simulink model "dyn_model"  (R2023b)
settings: Solver=VariableStepAuto  StartTime=0.0  StopTime=100.0  RelTol=1e-3
values from neighbouring files (symbols this model uses):
  A = double(A)    [dyn_model_mark.m]
  B = double(B)    [dyn_model_mark.m]
  C = [1 0 0 0 ... (first row only)    [dyn_model_mark.m]
  D = [0 ... (first row only)    [dyn_model_mark.m]
  g0 = 9.81    [dyn_model_mark.m]
  Ip = (mp*Lp^2)/12    (= 8.3205e-06)    [dyn_model_mark.m]
  Ir = (mr*(Lr/2)^2)/12    (= 1.42994791667e-05)    [dyn_model_mark.m]
  J = 4e-6    (= 4e-06)    [dyn_model_mark.m]
  k = 42e-3    (= 0.042)    [dyn_model_mark.m]
  La = 1.16e-3    (= 0.00116)    [dyn_model_mark.m]
  Lp = 0.129/2    (= 0.0645)    [dyn_model_mark.m]
  Lr = 0.085    [dyn_model_mark.m]
  mp = 0.024    [dyn_model_mark.m]
  mr = 0.095    [dyn_model_mark.m]
  param = [mr mp Lr Lp Ir Ip g0]'    [dyn_model_mark.m]
  Ra = 8.4    [dyn_model_mark.m]
undefined symbols (not defined in the file or in its folder): rot_pend
libraries: slpidlib x2, simulink_extras x2, simulink x2
settings Model: Creator=Mark  LastModifiedBy=Mark
settings OptimizationCC: BlockReduction=off  DefaultParameterBehavior=Inlined  BufferReuse=off

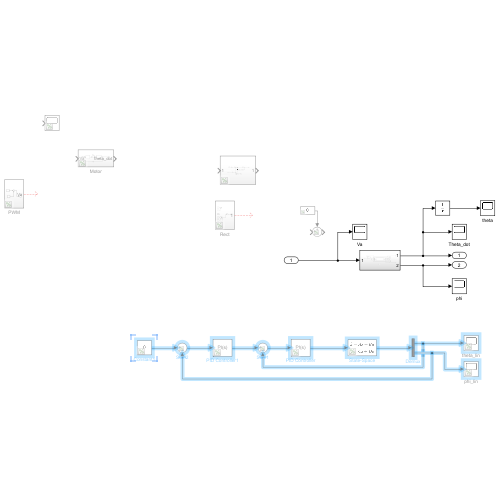
[thumbnail: Simulink's stored preview of the top-level diagram]
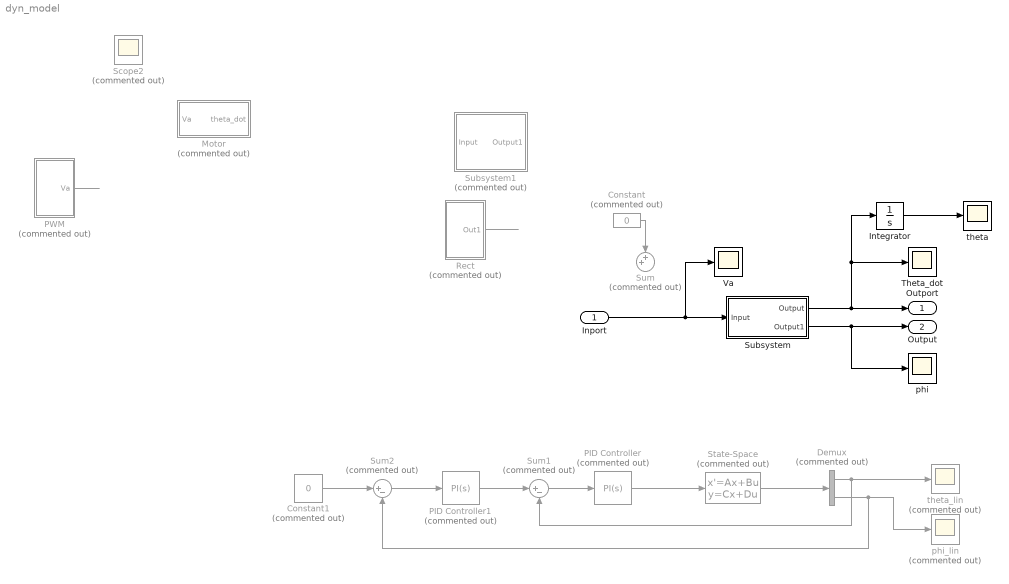
== system dyn_model ==
  Inport : Inport
  Constant : Constant  Commented=on  Value=0
  Constant1 : Constant  Commented=on  Value=0
  Demux : Demux  Commented=on  Outputs=2
  Integrator : Integrator
  Motor : Subsystem  Commented=on
  PID Controller : slpidlib/PID Controller  Commented=on  Controller=PI  Form=Parallel  TimeDomain=Continuous-time  UseExternalTs=off  SampleTime=-1  IntegratorMethod=Forward Euler  FilterMethod=Forward Euler  ControllerParametersSource=internal  P=1  I=1  UseKiTs=off  D=0  N=100  UseFilter=on  TunerSelectOption=Transfer Function Based (PID Tuner App)  InitialConditionSource=internal  InitialConditionForIntegrator=0  InitialConditionForFilter=0  DifferentiatorICPrevScaledInput=0  ExternalReset=none  TrackingMode=off  Kt=1  LimitOutput=off  SatLimitsSource=internal  UpperSaturationLimit=inf  LowerSaturationLimit=-inf  LinearizeAsGain=on  AntiWindupMode=none  Kb=1  LimitIntegrator=off  UpperIntegratorSaturationLimit=inf  LowerIntegratorSaturationLimit=-inf  POutMin=[]  POutMax=[]  IOutMin=[]  IOutMax=[]  DOutMin=[]  DOutMax=[]  NOutMin=[]  NOutMax=[]  SumOutMin=[]  SumOutMax=[]  SaturationOutMin=[]  SaturationOutMax=[]  PParamMin=[]  PParamMax=[]  IParamMin=[]  IParamMax=[]  DParamMin=[]  DParamMax=[]  NParamMin=[]  NParamMax=[]  KbParamMin=[]  KbParamMax=[]  KtParamMin=[]  KtParamMax=[]  KbOutMin=[]  KbOutMax=[]  KtOutMin=[]  KtOutMax=[]  IntegratorOutMin=[]  IntegratorOutMax=[]  FilterOutMin=[]  FilterOutMax=[]  SumI1OutMin=[]  SumI1OutMax=[]  SumI2OutMin=[]  SumI2OutMax=[]  SumI3OutMin=[]  SumI3OutMax=[]  SumI4OutMin=[]  SumI4OutMax=[]  SumDOutMin=[]  SumDOutMax=[]  DifferentiatorOutMin=[]  DifferentiatorOutMax=[]  FilterDiffOutCoefMin=[]  FilterDiffOutCoefMax=[]  ReciprocalOutMin=[]  ReciprocalOutMax=[]  SumDenOutMin=[]  SumDenOutMax=[]  SumNumOutMin=[]  SumNumOutMax=[]  DivideOutMin=[]  DivideOutMax=[]  UdiffTsProdOutMin=[]  UdiffTsProdOutMax=[]  NTsProdOutMin=[]  NTsProdOutMax=[]  UintegralTsProdOutMin=[]  UintegralTsProdOutMax=[]  UngainTsProdOutMin=[]  UngainTsProdOutMax=[]  ClampingZeroOutDataTypeStr=Inherit: Inherit via back propagation  ClampingZeroOutMin=[]  ClampingZeroOutMax=[]  FilterDenConstantOutDataTypeStr=Inherit: Inherit via back propagation  FilterDenConstantOutMin=[]  FilterDenConstantOutMax=[]  PCopyOutDataTypeStr=Inherit: Inherit via back propagation  PCopyOutMin=[]  PCopyOutMax=[]  NCopyOutDataTypeStr=Inherit: Inherit via back propagation  NCopyOutMin=[]  NCopyOutMax=[]  IntegratorContinuousStateAttributes=''  IntegratorStateMustResolveToSignalObject=off  IntegratorRTWStateStorageClass=Auto  FilterContinuousStateAttributes=''  FilterStateMustResolveToSignalObject=off  FilterRTWStateStorageClass=Auto  ParallelPVariant=InternalParameters  IdealPVariant=Disabled  IVariant=InternalParameters  DVariant=Disabled  IntegratorVariant=Continuous  SatVariant=Disabled  AWVariant=Passthrough  PCopyVariant=Disabled  TRVariant=Disabled  FdbkBlocksVariant=Forward  IdealPFdbkVariant=Disabled  SatFdbkVariant=Disabled  DerivativeFilterVariant=Disabled  NVariant=Disabled  NCopyVariant=Disabled_SignalSpec  FilterICVariant=Disabled  IntegratorICVariant=InternalICs  ExternalResetVariant=Disabled  TRSumVariant=Passthrough  SumFdbkVariant=Disabled  SumVariant=Sum_PI  TsampFilterVariant=InternalTs  TsampNgainVariant=Passthrough  TsampIntegralVariant=Disabled_SignalSpec  ExternalSaturationOutDataTypeStr=Inherit: Same as second input
  PID Controller1 : slpidlib/PID Controller  Commented=on  Controller=PI  Form=Parallel  TimeDomain=Continuous-time  UseExternalTs=off  SampleTime=-1  IntegratorMethod=Forward Euler  FilterMethod=Forward Euler  ControllerParametersSource=internal  P=1  I=1  UseKiTs=off  D=0  N=100  UseFilter=on  TunerSelectOption=Transfer Function Based (PID Tuner App)  InitialConditionSource=internal  InitialConditionForIntegrator=0  InitialConditionForFilter=0  DifferentiatorICPrevScaledInput=0  ExternalReset=none  TrackingMode=off  Kt=1  LimitOutput=off  SatLimitsSource=internal  UpperSaturationLimit=inf  LowerSaturationLimit=-inf  LinearizeAsGain=on  AntiWindupMode=none  Kb=1  LimitIntegrator=off  UpperIntegratorSaturationLimit=inf  LowerIntegratorSaturationLimit=-inf  POutMin=[]  POutMax=[]  IOutMin=[]  IOutMax=[]  DOutMin=[]  DOutMax=[]  NOutMin=[]  NOutMax=[]  SumOutMin=[]  SumOutMax=[]  SaturationOutMin=[]  SaturationOutMax=[]  PParamMin=[]  PParamMax=[]  IParamMin=[]  IParamMax=[]  DParamMin=[]  DParamMax=[]  NParamMin=[]  NParamMax=[]  KbParamMin=[]  KbParamMax=[]  KtParamMin=[]  KtParamMax=[]  KbOutMin=[]  KbOutMax=[]  KtOutMin=[]  KtOutMax=[]  IntegratorOutMin=[]  IntegratorOutMax=[]  FilterOutMin=[]  FilterOutMax=[]  SumI1OutMin=[]  SumI1OutMax=[]  SumI2OutMin=[]  SumI2OutMax=[]  SumI3OutMin=[]  SumI3OutMax=[]  SumI4OutMin=[]  SumI4OutMax=[]  SumDOutMin=[]  SumDOutMax=[]  DifferentiatorOutMin=[]  DifferentiatorOutMax=[]  FilterDiffOutCoefMin=[]  FilterDiffOutCoefMax=[]  ReciprocalOutMin=[]  ReciprocalOutMax=[]  SumDenOutMin=[]  SumDenOutMax=[]  SumNumOutMin=[]  SumNumOutMax=[]  DivideOutMin=[]  DivideOutMax=[]  UdiffTsProdOutMin=[]  UdiffTsProdOutMax=[]  NTsProdOutMin=[]  NTsProdOutMax=[]  UintegralTsProdOutMin=[]  UintegralTsProdOutMax=[]  UngainTsProdOutMin=[]  UngainTsProdOutMax=[]  ClampingZeroOutDataTypeStr=Inherit: Inherit via back propagation  ClampingZeroOutMin=[]  ClampingZeroOutMax=[]  FilterDenConstantOutDataTypeStr=Inherit: Inherit via back propagation  FilterDenConstantOutMin=[]  FilterDenConstantOutMax=[]  PCopyOutDataTypeStr=Inherit: Inherit via back propagation  PCopyOutMin=[]  PCopyOutMax=[]  NCopyOutDataTypeStr=Inherit: Inherit via back propagation  NCopyOutMin=[]  NCopyOutMax=[]  IntegratorContinuousStateAttributes=''  IntegratorStateMustResolveToSignalObject=off  IntegratorRTWStateStorageClass=Auto  FilterContinuousStateAttributes=''  FilterStateMustResolveToSignalObject=off  FilterRTWStateStorageClass=Auto  ParallelPVariant=InternalParameters  IdealPVariant=Disabled  IVariant=InternalParameters  DVariant=Disabled  IntegratorVariant=Continuous  SatVariant=Disabled  AWVariant=Passthrough  PCopyVariant=Disabled  TRVariant=Disabled  FdbkBlocksVariant=Forward  IdealPFdbkVariant=Disabled  SatFdbkVariant=Disabled  DerivativeFilterVariant=Disabled  NVariant=Disabled  NCopyVariant=Disabled_SignalSpec  FilterICVariant=Disabled  IntegratorICVariant=InternalICs  ExternalResetVariant=Disabled  TRSumVariant=Passthrough  SumFdbkVariant=Disabled  SumVariant=Sum_PI  TsampFilterVariant=InternalTs  TsampNgainVariant=Passthrough  TsampIntegralVariant=Disabled_SignalSpec  ExternalSaturationOutDataTypeStr=Inherit: Same as second input
  PWM : Subsystem  Commented=on
  Rect : Subsystem  Commented=on
  Scope2 : Scope  Commented=on
  State-Space : StateSpace  Commented=on  A=A  B=B  C=C  D=D  InitialCondition=0
  Subsystem : Subsystem
  Subsystem1 : Subsystem  Commented=on
  Sum : Sum  Commented=on  Inputs=++|
  Sum1 : Sum  Commented=on  Inputs=|+-
  Sum2 : Sum  Commented=on  Inputs=|+-
  Theta_dot : Scope
  Va : Scope
  phi : Scope
  phi_lin : Scope  Commented=on
  theta : Scope
  theta_lin : Scope  Commented=on
  Outport : Outport
  Output : Outport  Port=2
  wires:
  PWM/1(Va) -> ?
  Subsystem/1(Output) -> Outport/1, Integrator/1, Theta_dot/1
  Subsystem/2(Output1) -> phi/1, Output/1
  Inport/1 -> Va/1, Subsystem/1(Input)
  Integrator/1 -> theta/1
  Rect/1(Out1) -> ?
  Constant/1 -> Sum/1
  State-Space/1 -> Demux/1
  Demux/1 -> theta_lin/1, Sum1/2
  Demux/2 -> phi_lin/1, Sum2/2
  Sum2/1 -> PID Controller1/1
  Sum1/1 -> PID Controller/1
  PID Controller1/1 -> Sum1/1
  PID Controller/1 -> State-Space/1
  Constant1/1 -> Sum2/1

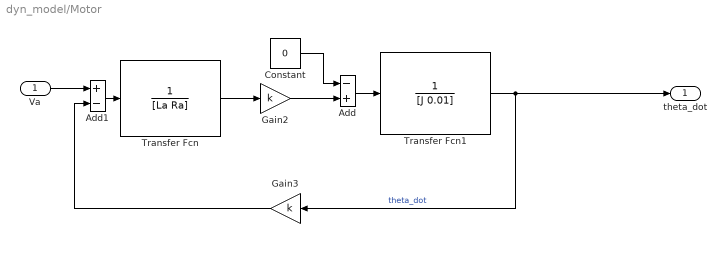
== system dyn_model/Motor ==
  Va : Inport
  Add : Sum  Inputs=-+
  Add1 : Sum  Inputs=+-
  Constant : Constant  Value=0
  Gain2 : Gain  Gain=k
  Gain3 : Gain  Gain=k
  Transfer Fcn : TransferFcn  Denominator=[La Ra]
  Transfer Fcn1 : TransferFcn  Denominator=[J 0.01]
  theta_dot : Outport
  wires:
  Gain3/1 -> Add1/2
  Transfer Fcn1/1 -> theta_dot/1, Gain3/1  "theta_dot"
  Add1/1 -> Transfer Fcn/1
  Va/1 -> Add1/1
  Constant/1 -> Add/1
  Gain2/1 -> Add/2
  Add/1 -> Transfer Fcn1/1
  Transfer Fcn/1 -> Gain2/1

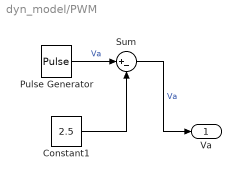
== system dyn_model/PWM ==
  Constant1 : Constant  Value=2.5
  Pulse Generator : DiscretePulseGenerator  PulseType=Time based  Amplitude=5  Period=10  PulseWidth=50
  Sum : Sum  Inputs=|+-
  Va : Outport
  wires:
  Pulse Generator/1 -> Sum/1  "Va"
  Constant1/1 -> Sum/2
  Sum/1 -> Va/1  "Va"

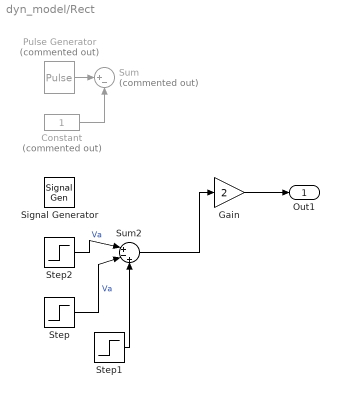
== system dyn_model/Rect ==
  Constant : Constant  Commented=on
  Gain : Gain  Gain=2
  Pulse Generator : DiscretePulseGenerator  Commented=on  PulseType=Time based  Amplitude=2  Period=1  PulseWidth=50  PhaseDelay=1
  Signal Generator : SignalGenerator  WaveForm=square  Amplitude=1.8  Frequency=0.5  Units=rad/sec
  Step : Step  Time=1.5  After=2  SampleTime=0
  Step1 : Step  Time=2  SampleTime=0
  Step2 : Step  SampleTime=0
  Sum : Sum  Commented=on  Inputs=|+-
  Sum2 : Sum  Inputs=|+-+
  Out1 : Outport
  wires:
  Step2/1 -> Sum2/1  "Va"
  Step/1 -> Sum2/2  "Va"
  Sum2/1 -> Gain/1
  Gain/1 -> Out1/1
  Constant/1 -> Sum/2
  Step1/1 -> Sum2/3
  Pulse Generator/1 -> Sum/1

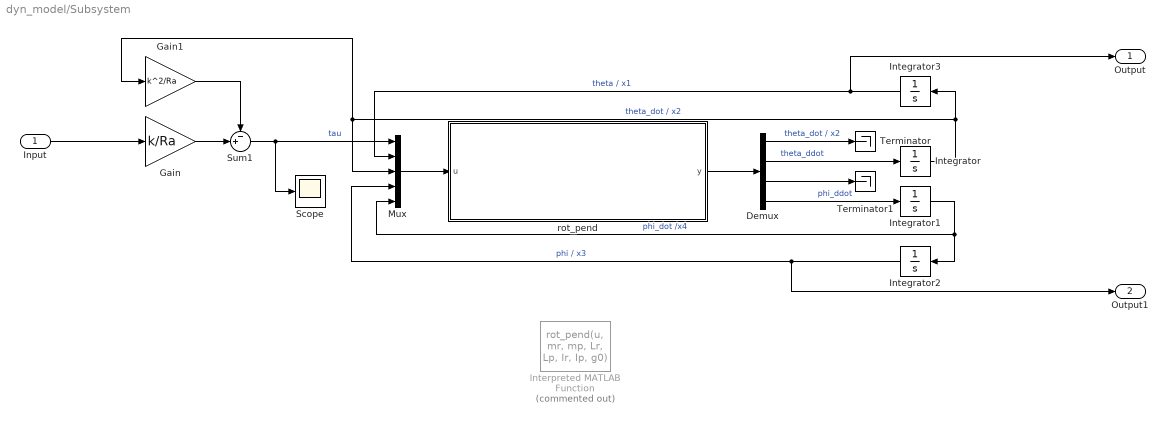
== system dyn_model/Subsystem ==
  Input : Inport
  Demux : Demux
  Gain : Gain  Gain=k/Ra
  Gain1 : Gain  Gain=k^2/Ra
  Integrator{,1..3} (4 alike) : Integrator
  Interpreted MATLAB Function : MATLABFcn  Commented=on  MATLABFcn=rot_pend(u, mr, mp, Lr, Lp, Ir, Ip, g0)  OutputDimensions=4  OutputSignalType=real
  Mux : Mux  Inputs=5
  Scope : Scope
  Sum1 : Sum  Inputs=-+|
  Terminator : Terminator
  Terminator1 : Terminator
  rot_pend : Subsystem
  Output : Outport
  Output1 : Outport  Port=2
  wires:
  Sum1/1 -> Scope/1, Mux/1  "tau"
  Integrator2/1 -> Output1/1, Mux/4  "phi / x3"
  Integrator/1 -> Integrator3/1, Gain1/1, Mux/3  "theta_dot / x2"
  Mux/1 -> rot_pend/1(u)
  rot_pend/1(y) -> Demux/1
  Gain/1 -> Sum1/2
  Integrator1/1 -> Mux/5, Integrator2/1  "phi_dot /x4"
  Gain1/1 -> Sum1/1
  Integrator3/1 -> Mux/2, Output/1  "theta / x1"
  Demux/4 -> Integrator1/1  "phi_ddot"
  Input/1 -> Gain/1
  Demux/2 -> Integrator/1  "theta_ddot"
  Demux/1 -> Terminator/1  "theta_dot / x2"
  Demux/3 -> Terminator1/1

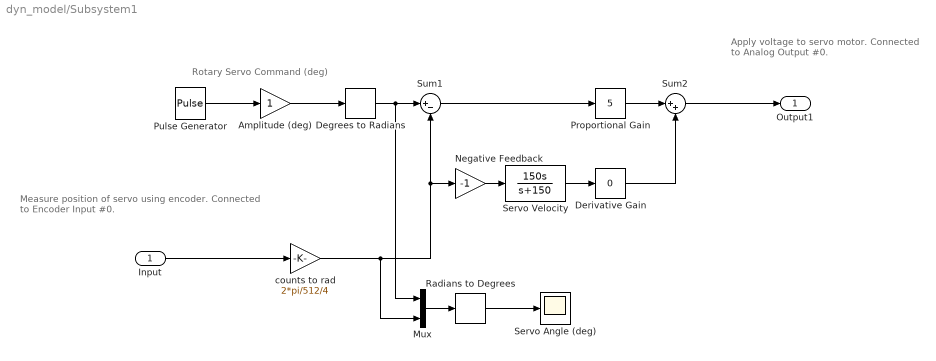
== system dyn_model/Subsystem1 ==
  note: Measure position of servo using encoder.
      | Connected to Encoder Input #0.
  note: Rotary Servo Command (deg)
  note: Apply voltage to servo motor.
      | Connected to Analog Output #0.
  Input : Inport
  Amplitude (deg) : Gain
  Degrees to Radians : simulink_extras/Transformations/Degrees to Radians
  Derivative Gain : simulink/Math Operations/Slider Gain  gain=0  low=0  high=0.5
  Mux : Mux  Inputs=2
  Negative Feedback : Gain  Gain=-1
  Proportional Gain : simulink/Math Operations/Slider Gain  gain=5  low=1  high=10
  Pulse Generator : DiscretePulseGenerator  PulseType=Time based  Amplitude=90  Period=10  PulseWidth=50
  Radians to Degrees : simulink_extras/Transformations/Radians to Degrees
  Servo Angle (deg) : Scope
  Servo Velocity : TransferFcn  Numerator=[150 0]  Denominator=[1 150]
  Sum1 : Sum  Inputs=|+-
  Sum2 : Sum  Inputs=|++
  counts to rad : Gain  Gain=2*pi/512/4
  Output1 : Outport
  wires:
  Negative Feedback/1 -> Servo Velocity/1
  Degrees to Radians/1 -> Sum1/1, Mux/1
  Amplitude (deg)/1 -> Degrees to Radians/1
  Derivative Gain/1 -> Sum2/2
  Servo Velocity/1 -> Derivative Gain/1
  Mux/1 -> Radians to Degrees/1
  Pulse Generator/1 -> Amplitude (deg)/1
  Sum1/1 -> Proportional Gain/1
  Radians to Degrees/1 -> Servo Angle (deg)/1
  counts to rad/1 -> Sum1/2, Negative Feedback/1, Mux/2
  Input/1 -> counts to rad/1
  Proportional Gain/1 -> Sum2/1
  Sum2/1 -> Output1/1

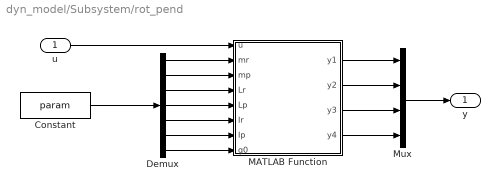
== system dyn_model/Subsystem/rot_pend ==
  u : Inport
  Constant : Constant  Value=param  VectorParams1D=off
  Demux : Demux  Outputs=7
  MATLAB Function : MATLAB Function  TreatAsAtomicUnit=on
  Mux : Mux
  y : Outport
  wires:
  Demux/3 -> MATLAB Function/4(Lr)
  Demux/5 -> MATLAB Function/6(Ir)
  Demux/4 -> MATLAB Function/5(Lp)
  Demux/7 -> MATLAB Function/8(g0)
  Demux/2 -> MATLAB Function/3(mp)
  Demux/6 -> MATLAB Function/7(Ip)
  Demux/1 -> MATLAB Function/2(mr)
  u/1 -> MATLAB Function/1(u)
  Constant/1 -> Demux/1
  MATLAB Function/1(y1) -> Mux/1
  MATLAB Function/2(y2) -> Mux/2
  MATLAB Function/3(y3) -> Mux/3
  MATLAB Function/4(y4) -> Mux/4
  Mux/1 -> y/1

== matlab function dyn_model/Subsystem/rot_pend/MATLAB Function ==
  data: u input; y1 output; mr input; mp input; Lr input; Lp input; Ir input; Ip input; g0 input; y2 output; y3 output; y4 output
function [y1,y2,y3,y4] = rot_pend(u, mr, mp, Lr, Lp, Ir, Ip, g0)
%UNTITLED Summary of this function goes here
%   Detailed explanation goes here
% u(1) = Va
x1 = u(2) ; % theta
x2 = u(3) ; % theta_dot
x3 = u(4) ; % phi
x4 = u(5) ; % phi_dot

a = mr*(Lr/2)^2 + mp*(Lr^2+(Lp*sin(x3))^2) + Ir ;
b = mp*Lr*Lp*cos(x3) ;
%c = b ;
d = mp*Lp^2+Ip ;

e = (-2*mp*Lp^2*sin(x3)*cos(x3)*x2*x4) + ( mp*Lr*Lp*sin(x3)*x2^2 ) + u(1) ;
f = ( mp*Lp^2*sin(x3)*cos(x3)*x2^2 ) + ( mp*g0*Lp*sin(x3) ) ;

B = [a b;
     b d] ;
ne = [e f]' ;
q_ddot = B\ne ;

y1 = x2 ;
y2 = q_ddot(1) ;
y3 = x4 ;
y4 = q_ddot(2) ;
